simulink model "sim"  (R2024b)
settings: Solver=VariableStepAuto  StartTime=0.0  StopTime=10.0  RelTol=1e-3
settings Model: Creator=Ishak  LastModifiedBy=Ishak

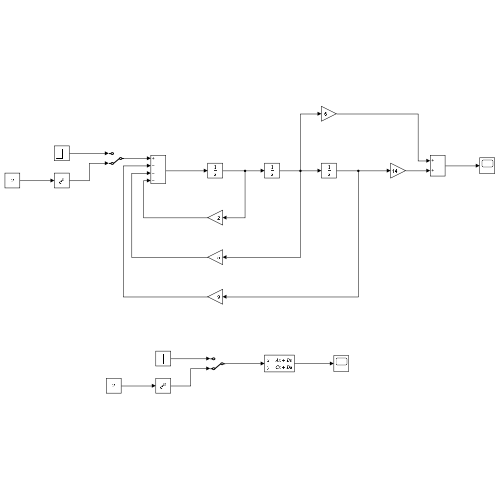
[thumbnail: Simulink's stored preview of the top-level diagram]
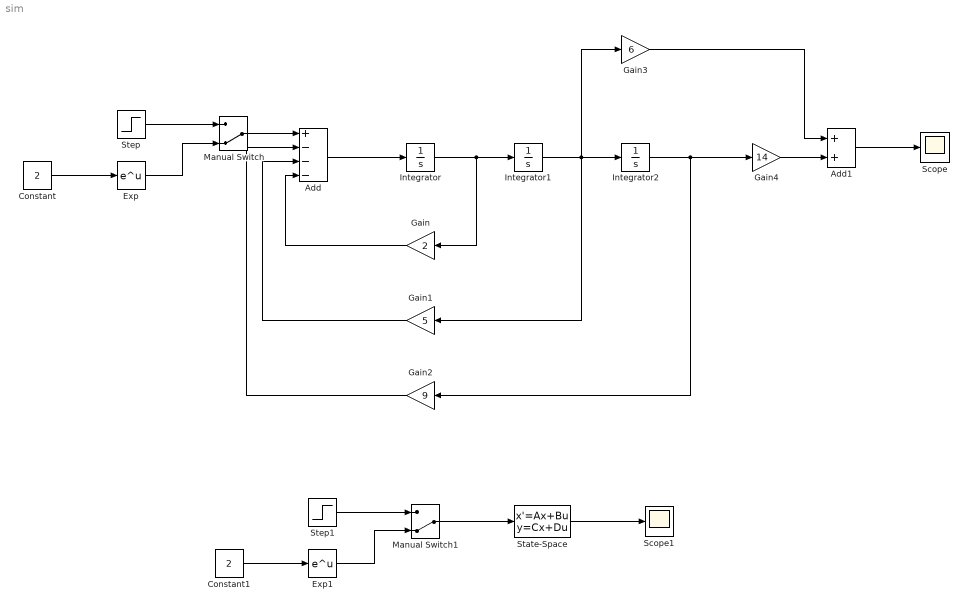
== system sim ==
  Add : Sum  Inputs=+---
  Add1 : Sum
  Constant : Constant  Value=2
  Constant1 : Constant  Value=2
  Exp : Math
  Exp1 : Math
  Gain : Gain  Gain=2
  Gain1 : Gain  Gain=5
  Gain2 : Gain  Gain=9
  Gain3 : Gain  Gain=6
  Gain4 : Gain  Gain=14
  Integrator : Integrator
  Integrator1 : Integrator
  Integrator2 : Integrator
  Manual Switch : ManualSwitch  CurrentSetting=0
  Manual Switch1 : ManualSwitch  CurrentSetting=0
  Scope : Scope
  Scope1 : Scope
  State-Space : StateSpace  A=[-2 -5 -9; 1 0 0; 0 1 0]  B=[1; 0; 0]  C="[0 6  14]"  D=0  InitialCondition=0
  Step : Step  SampleTime=0
  Step1 : Step  SampleTime=0
  wires:
  Add/1 -> Integrator/1
  Integrator/1 -> Gain/1, Integrator1/1
  Integrator1/1 -> Gain3/1, Gain1/1, Integrator2/1
  Step/1 -> Manual Switch/1
  Constant/1 -> Exp/1
  Exp/1 -> Manual Switch/2
  Manual Switch/1 -> Add/1
  Gain/1 -> Add/4
  Gain1/1 -> Add/3
  Integrator2/1 -> Gain2/1, Gain4/1
  Gain3/1 -> Add1/1
  Add1/1 -> Scope/1
  Gain4/1 -> Add1/2
  Gain2/1 -> Add/2
  Exp1/1 -> Manual Switch1/2
  Step1/1 -> Manual Switch1/1
  Constant1/1 -> Exp1/1
  Manual Switch1/1 -> State-Space/1
  State-Space/1 -> Scope1/1
